simulink model "model_stribeck_IC"  (R2023a)
settings: Solver=ode45  StartTime=0.0  StopTime=4  FixedStep=dt  MaxStep=0.001  RelTol=1e-3
values from neighbouring files (symbols this model uses):
  IC = [      0.2;      0.1*pi/180;      0;      0  ]    [program1.m]
settings Model: Creator=Adam  LastModifiedBy=Adam
settings SolverCC: AlgebraicLoopSolver=TrustRegion
settings DataIOCC: ExternalInput=ind  LoadExternalInput=on  SignalLogging=off  DSMLogging=off  OutputSaveName=out  ReturnWorkspaceOutputsName=sout
settings OptimizationCC: SimCompilerOptimization=on  AccelVerboseBuild=on
settings DebuggingCC: AlgebraicLoopMsg=none  UnconnectedInputMsg=warning  UnconnectedOutputMsg=warning  UnconnectedLineMsg=warning
settings ModelReferenceCC: EnableRefExpFcnMdlSchedulingChecks=on
settings RTWCC: DLArmComputeVersion=19.05

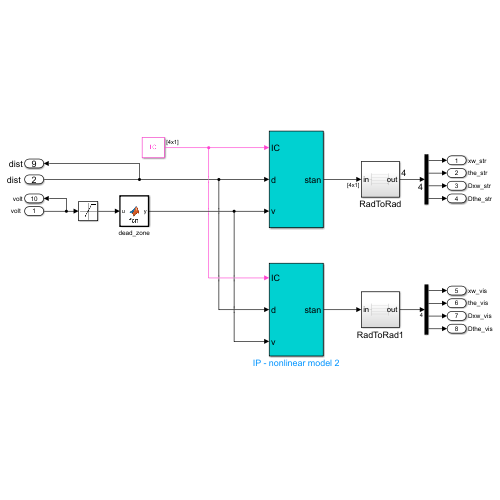
[thumbnail: Simulink's stored preview of the top-level diagram]
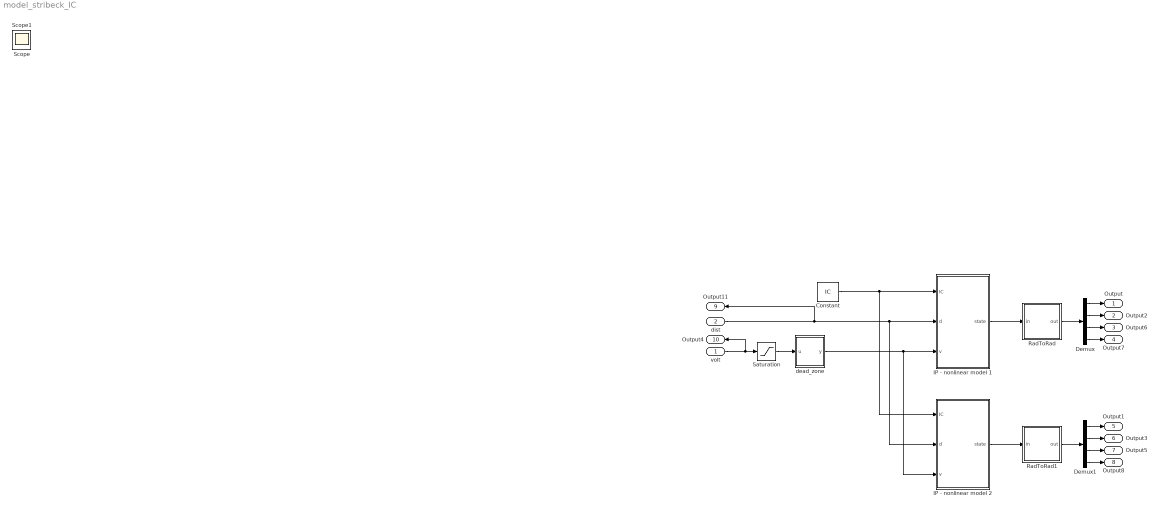
== system model_stribeck_IC ==
  volt : Inport
  dist : Inport  Port=2
  Constant : Constant  Value=IC  VectorParams1D=off
  Demux : Demux
  Demux1 : Demux
  IP - nonlinear model 1 : Subsystem  Description=Nonlinear model of inverted pendulum
      mask Display:
      | port_label('output', 1, 'stan');
      | port_label('input', 1, 'IC');
      | port_label('input', 2, 'd');
      | port_label('input', 3, 'v');
  IP - nonlinear model 2 : Subsystem  Description=Nonlinear model of inverted pendulum
      mask Display:
      | port_label('output', 1, 'stan');
      | port_label('input', 1, 'IC');
      | port_label('input', 2, 'd');
      | port_label('input', 3, 'v');
  RadToRad : Subsystem
  RadToRad1 : Subsystem
  Saturation : Saturate  UpperLimit=12  LowerLimit=-12
  dead_zone : MATLAB Function  TreatAsAtomicUnit=on
  Output : Outport  SignalName=xw_str
  Output2 : Outport  Port=2  SignalName=the_str
  Output6 : Outport  Port=3  SignalName=Dxw_str
  Output7 : Outport  Port=4  SignalName=Dthe_str
  Output1 : Outport  Port=5  SignalName=xw_vis
  Output3 : Outport  Port=6  SignalName=the_vis
  Output5 : Outport  Port=7  SignalName=Dxw_vis
  Output8 : Outport  Port=8  SignalName=Dthe_vis
  Output11 : Outport  Port=9  SignalName=dist
  Output4 : Outport  Port=10  SignalName=volt
  Scope : Scope
  Scope1 : Scope
  wires:
  IP - nonlinear model 1/1(state) -> RadToRad/1(in)
  Constant/1 -> IP - nonlinear model 1/1(IC), IP - nonlinear model 2/1(IC)
  dist/1 -> Output11/1, IP - nonlinear model 1/2(d), IP - nonlinear model 2/2(d)
  RadToRad/1(out) -> Demux/1
  volt/1 -> Output4/1, Saturation/1
  Demux/1 -> Output/1
  Demux/2 -> Output2/1
  Demux/3 -> Output6/1
  Demux/4 -> Output7/1
  Saturation/1 -> dead_zone/1(u)
  dead_zone/1(y) -> IP - nonlinear model 1/3(v), IP - nonlinear model 2/3(v)
  Demux1/2 -> Output3/1
  Demux1/3 -> Output5/1
  Demux1/1 -> Output1/1
  Demux1/4 -> Output8/1
  IP - nonlinear model 2/1(state) -> RadToRad1/1(in)
  RadToRad1/1(out) -> Demux1/1

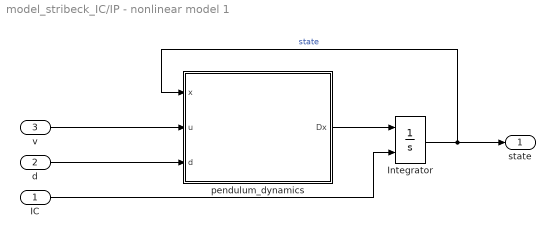
== system model_stribeck_IC/IP - nonlinear model 1 ==
  IC : Inport
  d : Inport  Port=2
  v : Inport  Port=3
  Integrator : Integrator  InitialConditionSource=external
  pendulum_dynamics : MATLAB Function  TreatAsAtomicUnit=on
  state : Outport
  wires:
  Integrator/1 -> state/1, pendulum_dynamics/1(x)  "state"
  v/1 -> pendulum_dynamics/2(u)
  pendulum_dynamics/1(Dx) -> Integrator/1
  IC/1 -> Integrator/2
  d/1 -> pendulum_dynamics/3(d)

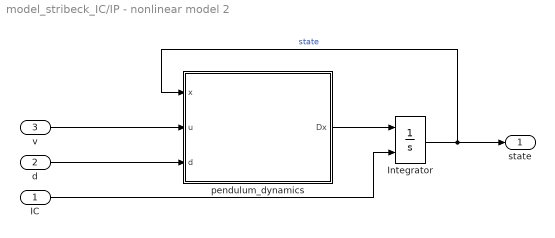
== system model_stribeck_IC/IP - nonlinear model 2 ==
  IC : Inport
  d : Inport  Port=2
  v : Inport  Port=3
  Integrator : Integrator  InitialConditionSource=external
  pendulum_dynamics : MATLAB Function  TreatAsAtomicUnit=on
  state : Outport
  wires:
  Integrator/1 -> state/1, pendulum_dynamics/1(x)  "state"
  v/1 -> pendulum_dynamics/2(u)
  pendulum_dynamics/1(Dx) -> Integrator/1
  IC/1 -> Integrator/2
  d/1 -> pendulum_dynamics/3(d)

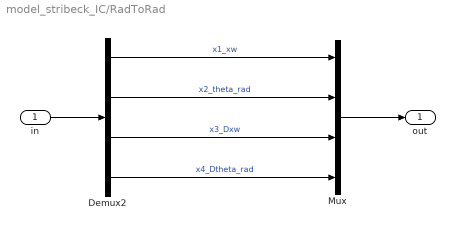
== system model_stribeck_IC/RadToRad ==
  in : Inport
  Demux2 : Demux
  Mux : Mux
  out : Outport
  wires:
  Demux2/1 -> Mux/1  "x1_xw"
  Demux2/2 -> Mux/2  "x2_theta_rad"
  in/1 -> Demux2/1
  Demux2/3 -> Mux/3  "x3_Dxw"
  Demux2/4 -> Mux/4  "x4_Dtheta_rad"
  Mux/1 -> out/1

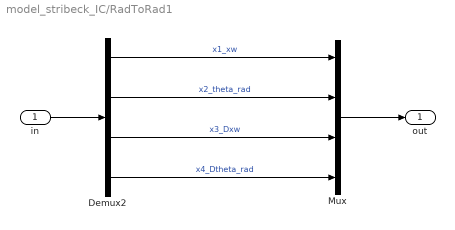
== system model_stribeck_IC/RadToRad1 ==
  in : Inport
  Demux2 : Demux
  Mux : Mux
  out : Outport
  wires:
  Demux2/1 -> Mux/1  "x1_xw"
  Demux2/2 -> Mux/2  "x2_theta_rad"
  in/1 -> Demux2/1
  Demux2/3 -> Mux/3  "x3_Dxw"
  Demux2/4 -> Mux/4  "x4_Dtheta_rad"
  Mux/1 -> out/1

== matlab function model_stribeck_IC/IP - nonlinear model 1/pendulum_dynamics ==
  data: x input; u input; d input; Dx output; params_strib parameter
function Dx = dynamika_wahadla(x, u, d, params_strib)
% x : stan
% u : input - napięcie
%
% params scope: "parameters"
%

% State, function input: x = [x Dx theta Dtheta]'
% x1 = x(1);
x2 = x(2);
x3 = x(3);
x4 = x(4);

params_strib = num2cell(params_strib);
[M, mp, mc, Lp, alpha_dcm, B, gamma_stri, miu_c, miu_s, vs] = params_strib{:};

g = 9.8145;
Lc = 2*Lp;
mr = mc + mp;
Mt = mr + M;
L = (Lc*mc + Lp*mp) / mr;
Jcm = 1/12*mp*Lp^2;
Jt = Jcm + mr*L^2;

i_i = 2;
delta_ = 600;

Ff = (miu_c + (miu_s-miu_c)*exp(-(x3/vs)^i_i)) * Mt*g*tanh(delta_*x3);
Fi = alpha_dcm*u;
A = d*cos(x2) - Ff + L*mr*x4^2*sin(x2) - B*x3 + Fi;
B = d*Lc + L*g*mr*sin(x2) - gamma_stri*x4;
DEN = Jt*Mt - (L*mr*cos(x2))^2;

ddt_x1 = x3;
ddt_x2 = x4;
ddt_x3 = (Jt*A - L*mr*cos(x2)*B) / DEN;
ddt_x4 = (Mt*B - L*mr*cos(x2)*A) / DEN;

% output
Dx = [ddt_x1 ddt_x2 ddt_x3 ddt_x4]';

end

== matlab function model_stribeck_IC/dead_zone ==
  data: u input; y output
function y = fcn(u)
    if (abs(u) < 1)
        y = 0;
    else
        y = u;
    end
end

== matlab function model_stribeck_IC/IP - nonlinear model 2/pendulum_dynamics ==
  data: x input; u input; d input; Dx output; params_vis parameter
function Dx = dynamika_wahadla(x, u, d, params_vis)
% x : stan
% u : input - napięcie
%
% params scope: "parameters"
%

% State, function input: x = [x Dx theta Dtheta]'
% x1 = x(1);
x2 = x(2);
x3 = x(3);
x4 = x(4);

params_vis = num2cell(params_vis);
[M, mp, mc, Lp, Bb, gamma_stri, alpha_dcm] = params_vis{:};

g = 9.8145;
Lc = 2*Lp;
mr = mc + mp;
Mt = mr + M;
L = (Lc*mc + Lp*mp) / mr;
Jcm = 1/12*mp*Lp^2;
Jt = Jcm + mr*L^2;

Fi = alpha_dcm*u;
A = d*cos(x2) + L*mr*x4^2*sin(x2) - Bb*x3 + Fi;
B = d*Lc + L*g*mr*sin(x2) - gamma_stri*x4;
DEN = Jt*Mt - (L*mr*cos(x2))^2;

ddt_x1 = x3;
ddt_x2 = x4;
ddt_x3 = (Jt*A - L*mr*cos(x2)*B) / DEN;
ddt_x4 = (Mt*B - L*mr*cos(x2)*A) / DEN;

% output
Dx = [ddt_x1 ddt_x2 ddt_x3 ddt_x4]';

end
